simulink model "SpacecraftOrientation"  (R2017b)
settings: Solver=ode4  StartTime=0.0  StopTime=1  FixedStep=0.01  RelTol=1e-3
settings Model: Creator=wol4aravio  LastModifiedBy=wol4aravio
settings DataIOCC: ExternalInput=[a, b]  SaveOutput=off  SignalLogging=off  DSMLogging=off  SaveTime=off

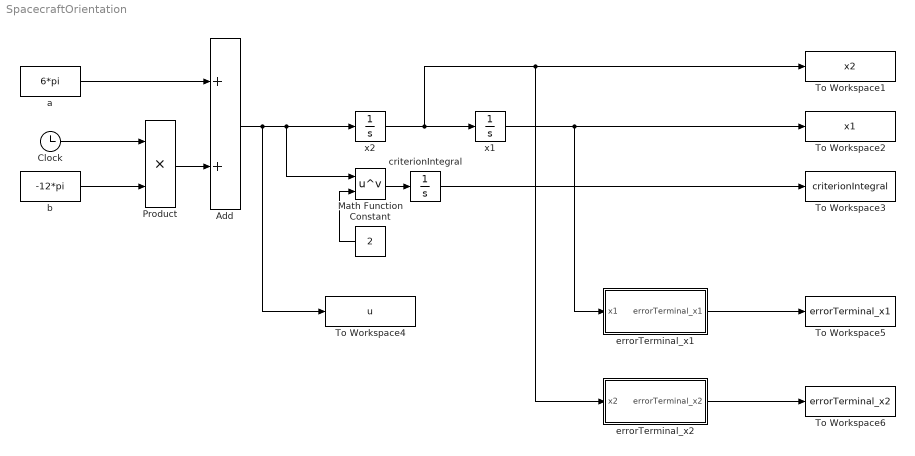
== system SpacecraftOrientation ==
  Add : Sum
  Clock : Clock
  Constant : Constant  Value=2
  Math Function : Math  Operator=pow  SaturateOnIntegerOverflow=on
  Product : Product
  To Workspace1 : ToWorkspace  VariableName=x2  SaveFormat=Timeseries  SampleTime=-1
  To Workspace2 : ToWorkspace  VariableName=x1  SaveFormat=Timeseries  SampleTime=-1
  To Workspace3 : ToWorkspace  VariableName=criterionIntegral  SaveFormat=Timeseries  SampleTime=-1
  To Workspace4 : ToWorkspace  VariableName=u  SaveFormat=Timeseries  SampleTime=-1
  To Workspace5 : ToWorkspace  VariableName=errorTerminal_x1  SaveFormat=Timeseries  SampleTime=-1
  To Workspace6 : ToWorkspace  VariableName=errorTerminal_x2  SaveFormat=Timeseries  SampleTime=-1
  a : Constant  Value=6*pi
  b : Constant  Value=-12*pi
  criterionIntegral : Integrator  ContinuousStateAttributes='criterionIntegral'
  errorTerminal_x1 : Subsystem
  errorTerminal_x2 : Subsystem
  x1 : Integrator  ContinuousStateAttributes='x1'
  x2 : Integrator  ContinuousStateAttributes='x2'
  wires:
  Clock/1 -> Product/1
  b/1 -> Product/2
  Product/1 -> Add/2
  a/1 -> Add/1
  Add/1 -> To Workspace4/1, Math Function/1, x2/1
  x2/1 -> errorTerminal_x2/1(x2), To Workspace1/1, x1/1
  Math Function/1 -> criterionIntegral/1
  Constant/1 -> Math Function/2
  criterionIntegral/1 -> To Workspace3/1
  errorTerminal_x2/1(errorTerminal_x2) -> To Workspace6/1
  errorTerminal_x1/1(errorTerminal_x1) -> To Workspace5/1
  x1/1 -> errorTerminal_x1/1(x1), To Workspace2/1

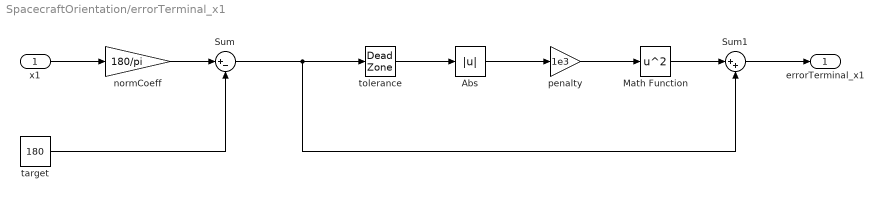
== system SpacecraftOrientation/errorTerminal_x1 ==
  x1 : Inport
  Abs : Abs
  Math Function : Math  Operator=square  SaturateOnIntegerOverflow=on
  Sum : Sum  Inputs=|+-
  Sum1 : Sum  Inputs=|++
  normCoeff : Gain  Gain=180/pi
  penalty : Gain  Gain=1e3
  target : Constant  Value=180
  tolerance : DeadZone  LowerValue=-1e-2  UpperValue=1e-2  SaturateOnIntegerOverflow=on
  errorTerminal_x1 : Outport
  wires:
  x1/1 -> normCoeff/1
  target/1 -> Sum/2
  tolerance/1 -> Abs/1
  Sum1/1 -> errorTerminal_x1/1
  Abs/1 -> penalty/1
  penalty/1 -> Math Function/1
  Math Function/1 -> Sum1/1
  Sum/1 -> Sum1/2, tolerance/1
  normCoeff/1 -> Sum/1

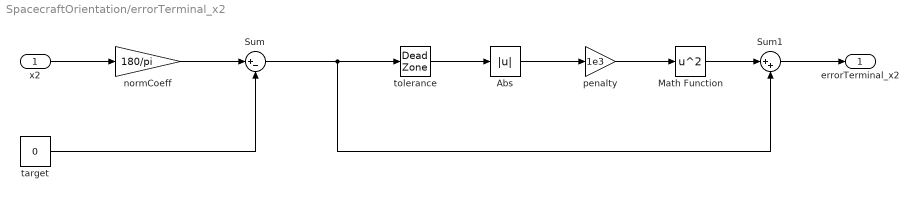
== system SpacecraftOrientation/errorTerminal_x2 ==
  x2 : Inport
  Abs : Abs
  Math Function : Math  Operator=square  SaturateOnIntegerOverflow=on
  Sum : Sum  Inputs=|+-
  Sum1 : Sum  Inputs=|++
  normCoeff : Gain  Gain=180/pi
  penalty : Gain  Gain=1e3
  target : Constant  Value=0
  tolerance : DeadZone  LowerValue=-1e-2  UpperValue=1e-2  SaturateOnIntegerOverflow=on
  errorTerminal_x2 : Outport
  wires:
  x2/1 -> normCoeff/1
  target/1 -> Sum/2
  tolerance/1 -> Abs/1
  Sum1/1 -> errorTerminal_x2/1
  Abs/1 -> penalty/1
  penalty/1 -> Math Function/1
  Math Function/1 -> Sum1/1
  Sum/1 -> Sum1/2, tolerance/1
  normCoeff/1 -> Sum/1
